simulink model "Transfer_function"  (R2024a)
settings: Solver=VariableStepAuto  StartTime=0.0  StopTime=10  RelTol=1e-3
values from neighbouring files (symbols this model uses):
  b = 0.1    [Constants.m]
  Cr1 = 0.075    [Constants.m]
  Cr1max = ke1*1.576    (= 0.5516)    [Constants.m]
  Cr2 = 0.069    [Constants.m]
  Cr2max = ke2*1.350    (= 0.486)    [Constants.m]
  f1 = 0.001    [Constants.m]
  f2 = 0.0003    [Constants.m]
  g = 9.81    [Constants.m]
  Jm1 = 0.0025    [Constants.m]
  Jm2 = 0.0027    [Constants.m]
  ke1 = 0.35    [Constants.m]
  ke2 = 0.36    [Constants.m]
  kt1 = ke1    (= 0.35)    [Constants.m]
  kt2 = ke2    (= 0.36)    [Constants.m]
  l = 14.94872e-3    (= 0.01494872)    [Constants.m]
  L1 = 2.8e-3    (= 0.0028)    [Constants.m]
  L2 = 2.9e-3    (= 0.0029)    [Constants.m]
  Lxx = 222.69522e-6    (= 0.00022269522)    [Constants.m]
  m = 0.52    [Constants.m]
  M = 2*0.011    (= 0.022)    [Constants.m]
  q = (M+m)*(Lxx+m*l^2)-(m*l)^2    (= 0.000123257240027)    [Constants.m]
  r = 42e-3    (= 0.042)    [Constants.m]
  R1 = 2.8    [Constants.m]
  R2 = 3.8    [Constants.m]
  Vmax = 6.00    (= 6)    [Constants.m]
undefined symbols (not defined in the file or in its folder): f, Jm, ke, kt, L, R, y
libraries: slpidlib x3
settings Model: PacingRate=0.010000  Creator=arthurtamboise  LastModifiedBy=arthurtamboise
settings RTWCC: GPUComputeCapability=3.5

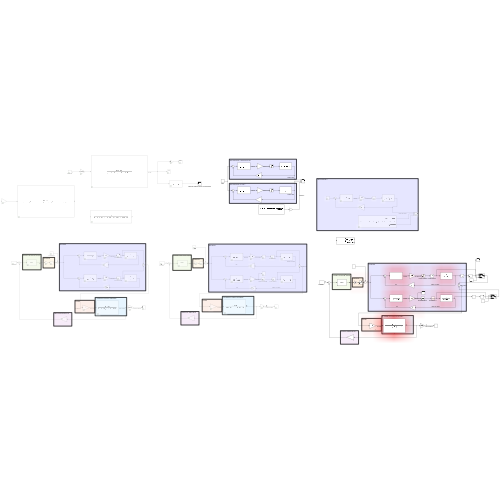
[thumbnail: Simulink's stored preview of the top-level diagram]
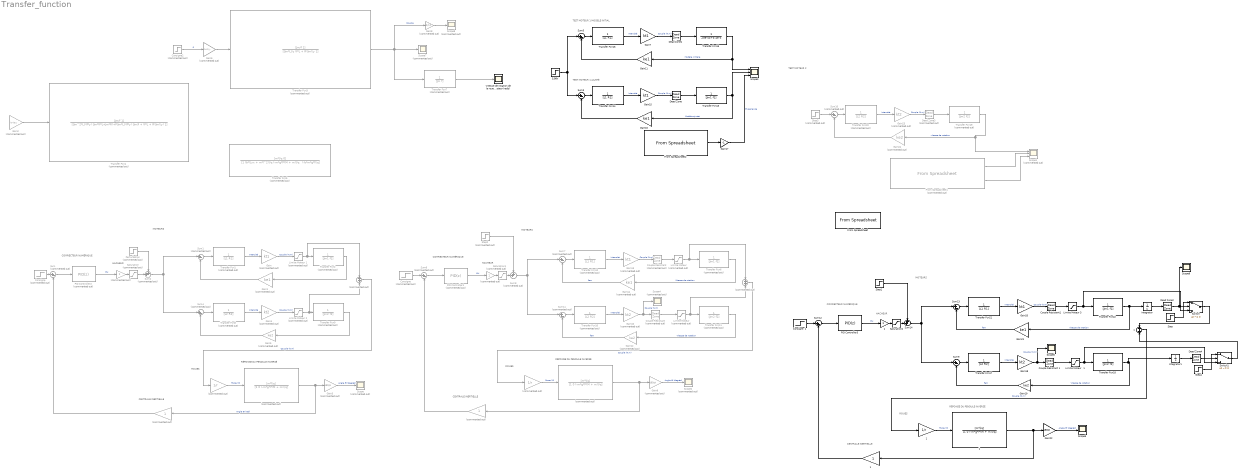
== system Transfer_function ==
  note: TEST MOTEUR 1 AJUSTÉ
  note: HACHEUR
  note: CENTRALE INERTIELLE
  note: CORRECTEUR NUMÉRIQUE
  note: MOTEURS
  note: RÉPONSE DU PENDULE INVERSÉ
  note: ROUES
  note: CORRECTEUR NUMÉRIQUE
  note: CENTRALE INERTIELLE
  note: MOTEURS
  note: ROUES
  note: RÉPONSE DU PENDULE INVERSÉ
  note: HACHEUR
  note: TEST MOTEUR 2
  note: TEST MOTEUR 1 MODELE INITIAL
  note: HACHEUR
  note: MOTEURS
  note: RÉPONSE DU PENDULE INVERSÉ
  note: ROUES
  note: CENTRALE INERTIELLE
  note: CORRECTEUR NUMÉRIQUE
  " " : Gain  Commented=on  Gain=1/r
  "  " : TransferFcn  Commented=on  Numerator=[m*l/q]  Denominator=[1 0 (-m*g*l*(M + m))/q]
  "   " : Sum  Commented=on  Inputs=+|+
  "       " : Gain  Commented=on
  "         " : Gain  Commented=on
  "          " : TransferFcn  Commented=on  Numerator=[m*l/q]  Denominator=[1 0 (-m*g*l*(M + m))/q]
  "                    " : Gain  Commented=on
  "                      " : Gain  Commented=on  Gain=1/r
  "                        " : Sum  Commented=on  Inputs=+|+
  "                           " : Gain  Commented=on
  "                           1" : Gain
  "                        1" : Sum  Inputs=+|+
  "                      1" : Gain  Gain=1/r
  "                    1" : Gain
  "  1" : TransferFcn  Numerator=[m*l/q]  Denominator=[1 0 (-m*g*l*(M + m))/q]
  5,98V : Step  Time=10  Before=5.98  After=0  SampleTime=0
  Consigne : Step  Commented=on  Time=0  After=0  SampleTime=0
  "Consigne  " : Step  Commented=on  Time=0  After=0  SampleTime=0
  Consigne  1 : Step  Time=0  After=0  SampleTime=0
  Consigne2 : Step  Commented=on  Time=0  Before=Vmax  After=Vmax  SampleTime=0
  Couple Résistant : DeadZone  Commented=on  LowerValue=-Cr1  UpperValue=Cr1
  "Couple Résistant " : DeadZone  Commented=on  LowerValue=-Cr2  UpperValue=Cr2
  Couple Résistant 1 : DeadZone  LowerValue=-Cr2  UpperValue=Cr2
  Couple Résistant1 : DeadZone  LowerValue=-Cr1  UpperValue=Cr1
  Dead Zone : DeadZone  LowerValue=-Cr1  UpperValue=Cr1
  Dead Zone1 : DeadZone  LowerValue=-Cr1  UpperValue=Cr1
  Dead Zone2 : DeadZone  LowerValue=-2.5/40  UpperValue=2.5/40
  Dead Zone3 : DeadZone  Commented=on  LowerValue=-Cr1  UpperValue=Cr1
  Dead Zone4 : DeadZone  LowerValue=-2.5/40  UpperValue=2.5/40
  From Spreadsheet : FromSpreadsheet  FileName=/Users/arthurtamboise/Desktop/TIPE/Constante_Vitesse_du_moteur/Vitesse_100_20_mot1.xlsx
  From Spreadsheet1 : FromSpreadsheet  Commented=on  FileName=/Users/arthurtamboise/Desktop/TIPE/Constante_Vitesse_du_moteur/Vitesse[100]_mot2.xlsx
  From Spreadsheet2 : FromSpreadsheet  FileName=/Users/arthurtamboise/Desktop/TIPE/Constante_Vitesse_du_moteur/Vitesse_100_20_mot1_2.xlsx  SheetName=in
  Gain : Gain  Commented=on  Gain=kt1
  Gain1 : Gain  Commented=on  Gain=ke1
  Gain10 : Gain  Commented=on  Gain=kt2
  Gain11 : Gain  Gain=ke1
  Gain12 : Gain  Commented=on  Gain=ke2
  Gain13 : Gain  Commented=on  Gain=kt1
  Gain14 : Gain  Commented=on  Gain=ke1
  Gain15 : Gain  Gain=kt1
  Gain16 : Gain  Gain=ke1
  Gain17 : Gain  Gain=-1
  Gain18 : Gain  Gain=kt2
  Gain19 : Gain  Gain=ke2
  Gain2 : Gain  Commented=on  Gain=kt*ke/y
  Gain20 : Gain  Gain=kt1
  Gain21 : Gain  Gain=ke1
  Gain22 : Gain  Gain=180/pi
  Gain23 : Gain  Commented=on  Gain=kt2
  Gain24 : Gain  Commented=on  Gain=ke2
  Gain3 : Gain  Commented=on  Gain=180/pi
  Gain4 : Gain  Commented=on  Gain=kt2
  Gain5 : Gain  Commented=on  Gain=ke2
  Gain6 : Gain  Commented=on  Gain=(kt*f)/y
  Gain7 : Gain  Gain=kt1
  Gain8 : Gain  Commented=on  Gain=1/kt
  Gain9 : Gain  Commented=on  Gain=180/pi
  Integrator : Integrator
  Integrator1 : Integrator
  "Limite Moteur " : Saturate  Commented=on  UpperLimit=Cr1max  LowerLimit=-Cr1max
  "Limite Moteur   " : Saturate  Commented=on  UpperLimit=Cr2max  LowerLimit=-Cr2max
  Limite Moteur   1 : Saturate  UpperLimit=Cr2max  LowerLimit=-Cr2max
  Limite Moteur 1 : Saturate  Commented=on  UpperLimit=Cr1max  LowerLimit=-Cr1max
  Limite Moteur 2 : Saturate  Commented=on  UpperLimit=Cr2max  LowerLimit=-Cr2max
  Limite Moteur 3 : Saturate  UpperLimit=Cr1max  LowerLimit=-Cr1max
  PID Controller1 : slpidlib/PID Controller  Commented=on  Controller=PID  Form=Parallel  TimeDomain=Discrete-time  UseExternalTs=off  SampleTime=0.015  IntegratorMethod=Backward Euler  FilterMethod=Backward Euler  ControllerParametersSource=internal  P=23  I=103  UseKiTs=off  D=0.67  UseExternalDerivativeSource=off  N=1000  UseFilter=on  TunerSelectOption=Transfer Function Based (PID Tuner App)  InitialConditionSource=internal  InitialConditionForIntegrator=0  InitialConditionForFilter=0  DifferentiatorICPrevScaledInput=0  ExternalReset=none  TrackingMode=off  Kt=1  LimitOutput=off  SatLimitsSource=internal  UpperSaturationLimit=Vmax  LowerSaturationLimit=-Vmax  LinearizeAsGain=off  AntiWindupMode=none  Kb=1  LimitIntegrator=off  UpperIntegratorSaturationLimit=inf  LowerIntegratorSaturationLimit=-inf  RndMeth=Nearest  POutMin=[]  POutMax=[]  IOutMin=[]  IOutMax=[]  DOutMin=[]  DOutMax=[]  NOutMin=[]  NOutMax=[]  SumOutMin=[]  SumOutMax=[]  SaturationOutMin=[]  SaturationOutMax=[]  PParamMin=[]  PParamMax=[]  IParamMin=[]  IParamMax=[]  DParamMin=[]  DParamMax=[]  NParamMin=[]  NParamMax=[]  KbParamMin=[]  KbParamMax=[]  KtParamMin=[]  KtParamMax=[]  KbOutMin=[]  KbOutMax=[]  KtOutMin=[]  KtOutMax=[]  IntegratorOutMin=[]  IntegratorOutMax=[]  FilterOutMin=[]  FilterOutMax=[]  SumI1OutMin=[]  SumI1OutMax=[]  SumI2OutMin=[]  SumI2OutMax=[]  SumI3OutMin=[]  SumI3OutMax=[]  SumI4OutMin=[]  SumI4OutMax=[]  SumDOutMin=[]  SumDOutMax=[]  DifferentiatorOutMin=[]  DifferentiatorOutMax=[]  FilterDiffOutCoefMin=[]  FilterDiffOutCoefMax=[]  ReciprocalOutMin=[]  ReciprocalOutMax=[]  SumDenOutMin=[]  SumDenOutMax=[]  SumNumOutMin=[]  SumNumOutMax=[]  DivideOutMin=[]  DivideOutMax=[]  UdiffTsProdOutMin=[]  UdiffTsProdOutMax=[]  NTsProdOutMin=[]  NTsProdOutMax=[]  UintegralTsProdOutMin=[]  UintegralTsProdOutMax=[]  UngainTsProdOutMin=[]  UngainTsProdOutMax=[]  ClampingZeroOutDataTypeStr=Inherit: Inherit via back propagation  ClampingZeroOutMin=[]  ClampingZeroOutMax=[]  FilterDenConstantOutDataTypeStr=Inherit: Inherit via back propagation  FilterDenConstantOutMin=[]  FilterDenConstantOutMax=[]  PCopyOutDataTypeStr=Inherit: Inherit via back propagation  PCopyOutMin=[]  PCopyOutMax=[]  NCopyOutDataTypeStr=Inherit: Inherit via back propagation  NCopyOutMin=[]  NCopyOutMax=[]  IntegratorContinuousStateAttributes=''  IntegratorStateMustResolveToSignalObject=off  IntegratorRTWStateStorageClass=Auto  FilterContinuousStateAttributes=''  FilterStateMustResolveToSignalObject=off  FilterRTWStateStorageClass=Auto  ParallelPVariant=InternalParameters  IdealPVariant=Disabled  IVariant=InternalParameters  DVariant=InternalParameters  IntegratorVariant=Discrete  SatVariant=Disabled  AWVariant=Passthrough  PCopyVariant=Disabled  TRVariant=Disabled  FdbkBlocksVariant=Forward  IdealPFdbkVariant=Disabled  SatFdbkVariant=Disabled  DerivativeFilterVariant=BackwardEulerFilter  NVariant=InternalParameters  NCopyVariant=InternalParameters  FilterICVariant=InternalICsFilter  IntegratorICVariant=InternalICs  ExternalResetVariant=Disabled  TRSumVariant=Passthrough  SumFdbkVariant=Disabled  SumVariant=Sum_PID  TsampFilterVariant=InternalTs  TsampNgainVariant=Passthrough  TsampIntegralVariant=Disabled_SignalSpec  ExternalSaturationOutDataTypeStr=Inherit: Same as second input  DerivativeSourceVariant=ErrorSignal
  PID Controller2 : slpidlib/PID Controller  Commented=on  Controller=PID  Form=Parallel  TimeDomain=Discrete-time  UseExternalTs=off  SampleTime=0.015  IntegratorMethod=Backward Euler  FilterMethod=Backward Euler  ControllerParametersSource=internal  P=23  I=103  UseKiTs=off  D=0.67  UseExternalDerivativeSource=off  N=5055.64703473953  UseFilter=off  TunerSelectOption=Transfer Function Based (PID Tuner App)  InitialConditionSource=internal  InitialConditionForIntegrator=0  InitialConditionForFilter=0  DifferentiatorICPrevScaledInput=0  ExternalReset=none  TrackingMode=off  Kt=1  LimitOutput=off  SatLimitsSource=internal  UpperSaturationLimit=Vmax  LowerSaturationLimit=-Vmax  LinearizeAsGain=off  AntiWindupMode=none  Kb=1  LimitIntegrator=off  UpperIntegratorSaturationLimit=inf  LowerIntegratorSaturationLimit=-inf  POutMin=[]  POutMax=[]  IOutMin=[]  IOutMax=[]  DOutMin=[]  DOutMax=[]  NOutMin=[]  NOutMax=[]  SumOutMin=[]  SumOutMax=[]  SaturationOutMin=[]  SaturationOutMax=[]  PParamMin=[]  PParamMax=[]  IParamMin=[]  IParamMax=[]  DParamMin=[]  DParamMax=[]  NParamMin=[]  NParamMax=[]  KbParamMin=[]  KbParamMax=[]  KtParamMin=[]  KtParamMax=[]  KbOutMin=[]  KbOutMax=[]  KtOutMin=[]  KtOutMax=[]  IntegratorOutMin=[]  IntegratorOutMax=[]  FilterOutMin=[]  FilterOutMax=[]  SumI1OutMin=[]  SumI1OutMax=[]  SumI2OutMin=[]  SumI2OutMax=[]  SumI3OutMin=[]  SumI3OutMax=[]  SumI4OutMin=[]  SumI4OutMax=[]  SumDOutMin=[]  SumDOutMax=[]  DifferentiatorOutMin=[]  DifferentiatorOutMax=[]  FilterDiffOutCoefMin=[]  FilterDiffOutCoefMax=[]  ReciprocalOutMin=[]  ReciprocalOutMax=[]  SumDenOutMin=[]  SumDenOutMax=[]  SumNumOutMin=[]  SumNumOutMax=[]  DivideOutMin=[]  DivideOutMax=[]  UdiffTsProdOutMin=[]  UdiffTsProdOutMax=[]  NTsProdOutMin=[]  NTsProdOutMax=[]  UintegralTsProdOutMin=[]  UintegralTsProdOutMax=[]  UngainTsProdOutMin=[]  UngainTsProdOutMax=[]  ClampingZeroOutDataTypeStr=Inherit: Inherit via back propagation  ClampingZeroOutMin=[]  ClampingZeroOutMax=[]  FilterDenConstantOutDataTypeStr=Inherit: Inherit via back propagation  FilterDenConstantOutMin=[]  FilterDenConstantOutMax=[]  PCopyOutDataTypeStr=Inherit: Inherit via back propagation  PCopyOutMin=[]  PCopyOutMax=[]  NCopyOutDataTypeStr=Inherit: Inherit via back propagation  NCopyOutMin=[]  NCopyOutMax=[]  IntegratorContinuousStateAttributes=''  IntegratorStateMustResolveToSignalObject=off  IntegratorRTWStateStorageClass=Auto  FilterContinuousStateAttributes=''  FilterStateMustResolveToSignalObject=off  FilterRTWStateStorageClass=Auto  ParallelPVariant=InternalParameters  IdealPVariant=Disabled  IVariant=InternalParameters  DVariant=InternalParameters  IntegratorVariant=Discrete  SatVariant=Disabled  AWVariant=Passthrough  PCopyVariant=Disabled  TRVariant=Disabled  FdbkBlocksVariant=Forward  IdealPFdbkVariant=Disabled  SatFdbkVariant=Disabled  DerivativeFilterVariant=Differentiator  NVariant=Passthrough  NCopyVariant=Disabled_SignalSpec  FilterICVariant=InternalICsDifferentiator  IntegratorICVariant=InternalICs  ExternalResetVariant=Disabled  TRSumVariant=Passthrough  SumFdbkVariant=Disabled  SumVariant=Sum_PID  TsampFilterVariant=InternalTs  TsampNgainVariant=Passthrough  TsampIntegralVariant=Disabled_SignalSpec  ExternalSaturationOutDataTypeStr=Inherit: Same as second input  DerivativeSourceVariant=ErrorSignal
  PID Controller3 : slpidlib/PID Controller  Controller=PID  Form=Parallel  TimeDomain=Discrete-time  UseExternalTs=off  SampleTime=0.015  IntegratorMethod=Backward Euler  FilterMethod=Backward Euler  ControllerParametersSource=internal  P=23  I=103  UseKiTs=off  D=0.67  UseExternalDerivativeSource=off  N=1000  UseFilter=on  TunerSelectOption=Transfer Function Based (PID Tuner App)  InitialConditionSource=internal  InitialConditionForIntegrator=0  InitialConditionForFilter=0  DifferentiatorICPrevScaledInput=0  ExternalReset=none  TrackingMode=off  Kt=1  LimitOutput=off  SatLimitsSource=internal  UpperSaturationLimit=Vmax  LowerSaturationLimit=-Vmax  LinearizeAsGain=off  AntiWindupMode=none  Kb=1  LimitIntegrator=off  UpperIntegratorSaturationLimit=inf  LowerIntegratorSaturationLimit=-inf  RndMeth=Nearest  POutMin=[]  POutMax=[]  IOutMin=[]  IOutMax=[]  DOutMin=[]  DOutMax=[]  NOutMin=[]  NOutMax=[]  SumOutMin=[]  SumOutMax=[]  SaturationOutMin=[]  SaturationOutMax=[]  PParamMin=[]  PParamMax=[]  IParamMin=[]  IParamMax=[]  DParamMin=[]  DParamMax=[]  NParamMin=[]  NParamMax=[]  KbParamMin=[]  KbParamMax=[]  KtParamMin=[]  KtParamMax=[]  KbOutMin=[]  KbOutMax=[]  KtOutMin=[]  KtOutMax=[]  IntegratorOutMin=[]  IntegratorOutMax=[]  FilterOutMin=[]  FilterOutMax=[]  SumI1OutMin=[]  SumI1OutMax=[]  SumI2OutMin=[]  SumI2OutMax=[]  SumI3OutMin=[]  SumI3OutMax=[]  SumI4OutMin=[]  SumI4OutMax=[]  SumDOutMin=[]  SumDOutMax=[]  DifferentiatorOutMin=[]  DifferentiatorOutMax=[]  FilterDiffOutCoefMin=[]  FilterDiffOutCoefMax=[]  ReciprocalOutMin=[]  ReciprocalOutMax=[]  SumDenOutMin=[]  SumDenOutMax=[]  SumNumOutMin=[]  SumNumOutMax=[]  DivideOutMin=[]  DivideOutMax=[]  UdiffTsProdOutMin=[]  UdiffTsProdOutMax=[]  NTsProdOutMin=[]  NTsProdOutMax=[]  UintegralTsProdOutMin=[]  UintegralTsProdOutMax=[]  UngainTsProdOutMin=[]  UngainTsProdOutMax=[]  ClampingZeroOutDataTypeStr=Inherit: Inherit via back propagation  ClampingZeroOutMin=[]  ClampingZeroOutMax=[]  FilterDenConstantOutDataTypeStr=Inherit: Inherit via back propagation  FilterDenConstantOutMin=[]  FilterDenConstantOutMax=[]  PCopyOutDataTypeStr=Inherit: Inherit via back propagation  PCopyOutMin=[]  PCopyOutMax=[]  NCopyOutDataTypeStr=Inherit: Inherit via back propagation  NCopyOutMin=[]  NCopyOutMax=[]  IntegratorContinuousStateAttributes=''  IntegratorStateMustResolveToSignalObject=off  IntegratorRTWStateStorageClass=Auto  FilterContinuousStateAttributes=''  FilterStateMustResolveToSignalObject=off  FilterRTWStateStorageClass=Auto  ParallelPVariant=InternalParameters  IdealPVariant=Disabled  IVariant=InternalParameters  DVariant=InternalParameters  IntegratorVariant=Discrete  SatVariant=Disabled  AWVariant=Passthrough  PCopyVariant=Disabled  TRVariant=Disabled  FdbkBlocksVariant=Forward  IdealPFdbkVariant=Disabled  SatFdbkVariant=Disabled  DerivativeFilterVariant=BackwardEulerFilter  NVariant=InternalParameters  NCopyVariant=InternalParameters  FilterICVariant=InternalICsFilter  IntegratorICVariant=InternalICs  ExternalResetVariant=Disabled  TRSumVariant=Passthrough  SumFdbkVariant=Disabled  SumVariant=Sum_PID  TsampFilterVariant=InternalTs  TsampNgainVariant=Passthrough  TsampIntegralVariant=Disabled_SignalSpec  ExternalSaturationOutDataTypeStr=Inherit: Same as second input  DerivativeSourceVariant=ErrorSignal
  Perturbation : Step  Commented=on  Time=0.001  Before=0.001  After=0  SampleTime=0
  Saturation : Saturate  Commented=on  UpperLimit=Vmax  LowerLimit=-Vmax
  Saturation1 : Saturate  Commented=on  UpperLimit=Vmax  LowerLimit=-Vmax
  Saturation2 : Saturate  UpperLimit=Vmax  LowerLimit=-Vmax
  Scope{,2,4,7..8} (5 alike) : Scope  Commented=on
  Scope1 : Scope  Commented=on  NumInputPorts=3
  Scope3 : Scope  NumInputPorts=3
  Scope5 : Scope
  Scope6 : Scope
  Scope9 : Scope
  Step : Step  Time=0  After=0  SampleTime=0
  Step1 : Step  Time=0.001  Before=10  After=0  SampleTime=0
  Step2 : Step  Commented=on  Time=0.001  Before=1  After=0  SampleTime=0
  Step3 : Step  Commented=on  Time=10  Before=6  After=0  SampleTime=0
  Step4 : Step  Time=0  After=0  SampleTime=0
  Sum{,1,4,6..7,10..11} (7 alike) : Sum  Commented=on  Inputs=|+-
  Sum{3,5,9,12..13} (5 alike) : Sum  Inputs=|+-
  Sum14 : Sum  Inputs=++|
  Sum2 : Sum  Commented=on  Inputs=++|
  Sum8 : Sum  Commented=on  Inputs=++|
  Switch : Switch  Criteria=u2 ~= 0  SaturateOnIntegerOverflow=off  InputSameDT=off
  Switch1 : Switch  Criteria=u2 ~= 0  SaturateOnIntegerOverflow=off  InputSameDT=off
  Transfer Fcn1 : TransferFcn  Commented=on  Denominator=[L1 R1]
  Transfer Fcn10 : TransferFcn  Commented=on  Denominator=[L2 R2]
  Transfer Fcn11 : TransferFcn  Commented=on  Denominator=[Jm2 f2]
  Transfer Fcn12 : TransferFcn  Commented=on  Denominator=[L1 R1]
  Transfer Fcn13 : TransferFcn  Denominator=[Jm1 f1]
  Transfer Fcn14 : TransferFcn  Denominator=[L1 R1]
  Transfer Fcn15 : TransferFcn  Denominator=[29e-5 9.4e-5]
  Transfer Fcn16 : TransferFcn  Denominator=[L1 R1]
  Transfer Fcn17 : TransferFcn  Denominator=[L2 R2]
  Transfer Fcn18 : TransferFcn  Denominator=[Jm2 f2]
  Transfer Fcn19 : TransferFcn  Commented=on  Denominator=[Jm2 f2]
  Transfer Fcn2 : TransferFcn  Commented=on  Denominator=[Jm1 f1]
  Transfer Fcn20 : TransferFcn  Commented=on  Denominator=[L2 R2]
  Transfer Fcn21 : TransferFcn  Denominator=[L1 R1]
  Transfer Fcn22 : TransferFcn  Denominator=[Jm1 f1]
  Transfer Fcn3 : TransferFcn  Commented=on  Numerator=[Jm/f 1]  Denominator=[(Jm*L)/y (f*L + R*Jm)/y 1]  ParameterTunability=Optimized
  Transfer Fcn4 : TransferFcn  Commented=on  Numerator=[Jm/f 1]  Denominator=[(Jm^2*L)/(f*y) (Jm*(f*L+Jm*R)+f*Jm*L)/(f*y) (Jm/f + (f*L + R*Jm)/y) 1]
  Transfer Fcn5 : TransferFcn  Commented=on  Numerator=[m*l/q 0]  Denominator="[1 (b*(Lxx + m*l^2))/q (-m*g*l*(M + m))/q   (-b*m*g*l)/q]"
  Transfer Fcn6 : TransferFcn  Commented=on  Denominator=[Jm1 f1]
  Transfer Fcn7 : TransferFcn  Commented=on  Denominator=[Jm f]
  Transfer Fcn8 : TransferFcn  Commented=on  Denominator=[L2 R2]
  Transfer Fcn9 : TransferFcn  Commented=on  Denominator=[Jm2 f2]
  Vitesse de rotation de la roue du moteur(rad/s) : Scope
  wires:
  Consigne/1 -> Sum/1
  Perturbation/1 -> Sum2/1
  Gain2/1 -> Transfer Fcn4/1
  Gain3/1 -> Scope/1  "Angle Θ (degrés)"
  Consigne2/1 -> Gain6/1  "0"
  Gain6/1 -> Transfer Fcn3/1
  Transfer Fcn3/1 -> Gain8/1, Transfer Fcn7/1, Scope7/1  "Couple"
  Transfer Fcn7/1 -> Vitesse de rotation de la roue du moteur(rad/s)/1
  Gain8/1 -> Scope8/1
  PID Controller2/1 -> "       "/1  "MLI"
  "          "/1 -> Gain3/1, "         "/1  "Angle Θ (rad)"
  "   "/1 -> " "/1  "Couple (N.m)"
  " "/1 -> "          "/1  "Force (N)"
  Sum4/1 -> Transfer Fcn8/1
  Sum2/1 -> Sum4/1, Sum1/1
  Gain4/1 -> Limite Moteur 2/1  "Couple (N.m)"
  Transfer Fcn1/1 -> Gain/1  "Intensité"
  Transfer Fcn8/1 -> Gain4/1  "Intensité"
  Gain5/1 -> Sum4/2
  Limite Moteur 1/1 -> Transfer Fcn2/1, "   "/1
  Transfer Fcn9/1 -> Gain5/1
  Gain/1 -> Limite Moteur 1/1  "Couple (N.m)"
  Limite Moteur 2/1 -> "   "/2, Transfer Fcn9/1
  Transfer Fcn2/1 -> Gain1/1
  Sum1/1 -> Transfer Fcn1/1
  Gain1/1 -> Sum1/2
  "         "/1 -> Sum/2
  Sum/1 -> PID Controller2/1
  Saturation/1 -> Sum2/2
  "       "/1 -> Saturation/1
  Transfer Fcn13/1 -> Scope3/2, Gain16/1  "Modèle ajusté"
  Gain16/1 -> Sum3/2
  Transfer Fcn14/1 -> Gain15/1  "Intensité"
  Sum3/1 -> Transfer Fcn14/1
  Gain15/1 -> Dead Zone/1  "Couple (N.m)"
  Dead Zone/1 -> Transfer Fcn13/1
  Gain9/1 -> Scope2/1  "Angle Θ (degrés)"
  "Consigne  "/1 -> Sum6/1
  Gain12/1 -> Sum11/2  "fem"
  Gain10/1 -> Scope4/1, "Couple Résistant "/1  "Couple (N.m)"
  "                        "/1 -> "                      "/1  "Couple (N.m)"
  Gain14/1 -> Sum7/2  "fem"
  "                           "/1 -> Sum6/2
  Sum8/1 -> Sum11/1, Sum7/1
  Couple Résistant/1 -> "Limite Moteur "/1
  Sum11/1 -> Transfer Fcn10/1
  Transfer Fcn12/1 -> Gain13/1  "Intensité"
  "                      "/1 -> "  "/1  "Force (N)"
  Step2/1 -> Sum8/1
  Transfer Fcn10/1 -> Gain10/1  "Intensité"
  Transfer Fcn6/1 -> Gain14/1  "Vitesse de rotation"
  "Limite Moteur   "/1 -> "                        "/2, Transfer Fcn11/1
  Sum7/1 -> Transfer Fcn12/1
  Gain13/1 -> Couple Résistant/1  "Couple (N.m)"
  Transfer Fcn11/1 -> Gain12/1  "Vitesse de rotation"
  "Limite Moteur "/1 -> Transfer Fcn6/1, "                        "/1
  Sum6/1 -> PID Controller1/1
  "Couple Résistant "/1 -> "Limite Moteur   "/1
  Transfer Fcn20/1 -> Gain23/1  "Intensité"
  Gain24/1 -> Sum10/2
  Transfer Fcn19/1 -> Scope1/1, Gain24/1  "vitesse de rotation"
  Step3/1 -> Sum10/1
  Sum10/1 -> Transfer Fcn20/1
  From Spreadsheet1/2 -> Scope1/3
  From Spreadsheet1/1 -> Scope1/2
  Gain23/1 -> Dead Zone3/1  "Couple (N.m)"
  Dead Zone3/1 -> Transfer Fcn19/1
  From Spreadsheet2/1 -> Gain17/1
  Saturation1/1 -> Sum8/2
  "                    "/1 -> Saturation1/1
  PID Controller1/1 -> "                    "/1  "MLI"
  Transfer Fcn16/1 -> Gain7/1  "Intensité"
  Gain11/1 -> Sum5/2
  5,98V/1 -> Sum5/1, Sum3/1
  Transfer Fcn15/1 -> Scope3/1, Gain11/1  "Modèle initiale"
  Sum5/1 -> Transfer Fcn16/1
  Dead Zone1/1 -> Transfer Fcn15/1
  Gain7/1 -> Dead Zone1/1  "Couple (N.m)"
  Gain17/1 -> Scope3/3  "Expérience"
  "  "/1 -> Gain9/1, "                           "/1
  Sum13/1 -> Transfer Fcn21/1
  Gain18/1 -> Scope6/1, Couple Résistant 1/1  "Couple (N.m)"
  Gain22/1 -> Scope5/1  "Angle Θ (degrés)"
  Gain20/1 -> Couple Résistant1/1  "Couple (N.m)"
  "                        1"/1 -> "                      1"/1  "Couple (N.m)"
  Gain19/1 -> Sum9/2  "fem"
  "                    1"/1 -> Saturation2/1
  Couple Résistant 1/1 -> Limite Moteur   1/1
  "  1"/1 -> Gain22/1, "                           1"/1
  Gain21/1 -> Sum13/2  "fem"
  Sum12/1 -> PID Controller3/1
  PID Controller3/1 -> "                    1"/1  "MLI"
  Consigne  1/1 -> Sum12/1
  Sum14/1 -> Sum9/1, Sum13/1
  "                      1"/1 -> "  1"/1  "Force (N)"
  "                           1"/1 -> Sum12/2
  Sum9/1 -> Transfer Fcn17/1
  Transfer Fcn17/1 -> Gain18/1  "Intensité"
  Step1/1 -> Sum14/1
  Transfer Fcn21/1 -> Gain20/1  "Intensité"
  Transfer Fcn18/1 -> Integrator1/1, Gain19/1  "Vitesse de rotation"
  Transfer Fcn22/1 -> Gain21/1, Integrator/1  "Vitesse de rotation"
  Limite Moteur 3/1 -> Switch/3, Transfer Fcn22/1
  Limite Moteur   1/1 -> Switch1/3, Transfer Fcn18/1
  Couple Résistant1/1 -> Limite Moteur 3/1
  Saturation2/1 -> Sum14/2
  Integrator/1 -> Dead Zone2/1
  Dead Zone2/1 -> Scope9/1, Switch/2
  Switch/1 -> "                        1"/1
  Dead Zone4/1 -> Switch1/2
  Integrator1/1 -> Dead Zone4/1
  Switch1/1 -> "                        1"/2
  Step/1 -> Switch/1
  Step4/1 -> Switch1/1
